simulink model "c960x4096_x14_7_r2013b_frb"  (R2013b)
settings: Solver=ode45  StartTime=0.0  StopTime=40960  RelTol=1e-3
undefined symbols (not defined in the file): sfp
libraries: xbsIndex_r4 x14620, casper_library_misc x61, dspsigops x32, casper_library_multipliers x24, simulink x18, xps_library x18
(part 36 of 79)

== system c960x4096_x14_7_r2013b_frb/ds_to_tgbe/mb_rd/XFER_5/GEN_R_ADDR_MUX_SEL ==
  MSYNC : Inport
  WE : Inport  Port=2
  NCHAN : Inport  Port=3
  9_bit_cntr : xbsIndex_r4/Counter  cnt_type=Free Running  cnt_to=Inf  operation=Up  start_count=0  cnt_by_val=1  arith_type=Unsigned  n_bits=9  bin_pt=0  load_pin=off  rst=on  en=on  explicit_period=on  period=1  dbl_ovrd=off  use_behavioral_HDL=off  implementation=Fabric  block_type=counter
  Concat : xbsIndex_r4/Concat  num_inputs=2  dbl_ovrd=off  block_type=concat
  DELAY_SEL : Subsystem
  Delay : xbsIndex_r4/Delay  rst=off  infoeditControl=Selection of Reset will increase slice count due to use of real FFs and instead of SRLs  en=off  latency=1  dbl_ovrd=off  reg_retiming=off  block_type=delay
  Logical : xbsIndex_r4/Logical  logical_function=OR  inputs=2  en=off  latency=0  precision=Full  arith_type=Unsigned  n_bits=16  bin_pt=0  align_bp=on  dbl_ovrd=off  block_type=logical
  Logical1 : xbsIndex_r4/Logical  logical_function=OR  inputs=2  en=off  latency=0  precision=Full  arith_type=Unsigned  n_bits=16  bin_pt=0  align_bp=on  dbl_ovrd=off  block_type=logical
  Logical2 : xbsIndex_r4/Logical  logical_function=OR  inputs=2  en=off  latency=0  precision=Full  arith_type=Unsigned  n_bits=16  bin_pt=0  align_bp=on  dbl_ovrd=off  block_type=logical
  Pad_3_MSBs : xbsIndex_r4/Constant  const=0  gui_display_data_type=Fixed-point  arith_type=Unsigned  n_bits=3  bin_pt=0  preci_type=Single  exp_width=8  frac_width=24  explicit_period=on  period=1  equ=P=C  opselect=C  inp2=PCIN>>17  opr=+  inp1=P  carry=CIN  dbl_ovrd=off  block_type=constant
  Register : xbsIndex_r4/Register  init=0  rst=on  en=off  dbl_ovrd=off  block_type=register
  Relational : xbsIndex_r4/Relational  mode=a=b  en=off  latency=0  dbl_ovrd=off  block_type=relational
  Slice_2_LSBs : xbsIndex_r4/Slice  nbits=2  boolean_output=off  mode=Lower Bit Location + Width  bit1=0  base1=MSB of Input  bit0=0  base0=LSB of Input  dbl_ovrd=off  block_type=slice
  Slice_7_MSBs : xbsIndex_r4/Slice  nbits=7  boolean_output=off  mode=Upper Bit Location + Width  bit1=0  base1=MSB of Input  bit0=0  base0=LSB of Input  dbl_ovrd=off  block_type=slice
  TERM_CNT : Subsystem
  edge_detect : Subsystem  AncestorBlock=casper_library_misc/edge_detect  mask(edge_detect){edge=Rising, polarity=Active High, x_in=[0 0.08 0.08 0.16 0.16 0.24 0.24 0.32 0.32 0.4], y_in=[-1 -1  1  1  1  1  1  1  1  1], x_out=[0.6 0.68 0.68 0.76 0.76 0.84 0.84 0.92 0.92 1], y_out=[-1 -1  1  1 -1 -1 -1 -1 -1 -1]}
      mask prompts: edge "Edge Type"; polarity "Output Polarity"; x_in "Input X Positions"; y_in "Input Y Positions"; x_out "Output X Positions"; y_out "Output Y Positions"
      mask help: Output is active for one-cycle after each edge of the specified type (i.e. rising, falling or both).
      mask init: same as c960x4096_x14_7_r2013b_frb/edge_detect2
      settings: AttributesFormatString=|
      | rising edges
      | active high
      mask Help: Output is active for one-cycle after each edge of the specified type (i.e. rising, falling, or both).  Latency is zero.
      mask TypeOptions edge: Rising | Falling | Both
      mask TypeOptions polarity: Active High | Active Low
      mask Display:
      | plot(x_in_num,0.5+y_in_num*0.2);
      | plot(x_out_num,0.5+y_out_num*0.2);
  R_ADDR : Outport
  MUX_SEL : Outport  Port=2
  wires:
  DELAY_SEL/1(TRIG) -> Logical/2
  edge_detect/1(out) -> DELAY_SEL/2(WE_PE)
  [NCHAN] -> DELAY_SEL/1(NCHAN)
  [WE] -> edge_detect/1(in)
  [MSYNC] -> Logical2/2
  Logical2/1 -> Register/2
  Register/1 -> 9_bit_cntr/2, Logical/1
  Logical/1 -> Register/1
  Delay/1 -> MUX_SEL/1
  NCHAN/1 -> [NCHAN]
  WE/1 -> [WE]
  MSYNC/1 -> [MSYNC]
  Slice_2_LSBs/1 -> Delay/1
  Concat/1 -> R_ADDR/1
  Relational/1 -> Logical1/1, Logical2/1
  Slice_7_MSBs/1 -> Concat/2
  Pad_3_MSBs/1 -> Concat/1
  [NCHAN] -> TERM_CNT/1(NCHAN)
  TERM_CNT/1(OUT) -> Relational/2
  [MSYNC] -> Logical1/2
  Logical1/1 -> 9_bit_cntr/1
  9_bit_cntr/1 -> Slice_7_MSBs/1, Slice_2_LSBs/1, Relational/1

== system c960x4096_x14_7_r2013b_frb/ds_to_tgbe/mb_rd/XFER_5/GEN_STB_EOF_W_COUNT ==
  MSYNC : Inport
  WE : Inport  Port=2
  NCHAN : Inport  Port=3
  2_RST : xbsIndex_r4/Constant  const=1027  gui_display_data_type=Fixed-point  arith_type=Unsigned  n_bits=11  bin_pt=0  preci_type=Single  exp_width=8  frac_width=24  explicit_period=on  period=1  equ=P=C  opselect=C  inp2=PCIN>>17  opr=+  inp1=P  carry=CIN  dbl_ovrd=off  block_type=constant
  A_LENGTH : Subsystem
  AddSub : xbsIndex_r4/AddSub  mode=Addition  use_carryin=off  use_carryout=off  en=off  latency=0  precision=Full  arith_type=Unsigned  n_bits=16  bin_pt=14  quantization=Truncate  overflow=Wrap  dbl_ovrd=off  use_behavioral_HDL=off  hw_selection=Fabric  pipelined=off  block_type=addsub
  B_LENGTH : Subsystem
  C_LENGTH : Subsystem
  Convert : xbsIndex_r4/Convert  gui_display_data_type=Fixed-point  arith_type=Unsigned  n_bits=1  bin_pt=0  float_type=Single  exp_bits=8  fraction_bits=24  quantization=Truncate  overflow=Wrap  en=off  latency=0  dbl_ovrd=off  pipeline=off  block_type=convert
  Convert1 : xbsIndex_r4/Convert  gui_display_data_type=Fixed-point  arith_type=Unsigned  n_bits=1  bin_pt=0  float_type=Single  exp_bits=8  fraction_bits=24  quantization=Truncate  overflow=Wrap  en=off  latency=0  dbl_ovrd=off  pipeline=off  block_type=convert
  Counter : xbsIndex_r4/Counter  cnt_type=Free Running  cnt_to=Inf  operation=Up  start_count=0  cnt_by_val=1  arith_type=Unsigned  n_bits=11  bin_pt=0  load_pin=off  rst=on  en=on  explicit_period=on  period=1  dbl_ovrd=off  use_behavioral_HDL=off  implementation=Fabric  block_type=counter
  Delay : xbsIndex_r4/Delay  rst=off  infoeditControl=Selection of Reset will increase slice count due to use of real FFs and instead of SRLs  en=off  latency=0  dbl_ovrd=off  reg_retiming=off  block_type=delay
  Delay1 : xbsIndex_r4/Delay  rst=off  infoeditControl=Selection of Reset will increase slice count due to use of real FFs and instead of SRLs  en=off  latency=1  dbl_ovrd=off  reg_retiming=off  block_type=delay
  Delay2 : xbsIndex_r4/Delay  rst=off  infoeditControl=Selection of Reset will increase slice count due to use of real FFs and instead of SRLs  en=off  latency=1  dbl_ovrd=off  reg_retiming=off  block_type=delay
  Delay3 : xbsIndex_r4/Delay  rst=off  infoeditControl=Selection of Reset will increase slice count due to use of real FFs and instead of SRLs  en=off  latency=2  dbl_ovrd=off  reg_retiming=off  block_type=delay
  Delay4 : xbsIndex_r4/Delay  rst=off  infoeditControl=Selection of Reset will increase slice count due to use of real FFs and instead of SRLs  en=off  latency=2  dbl_ovrd=off  reg_retiming=off  block_type=delay
  Delay5 : xbsIndex_r4/Delay  rst=off  infoeditControl=Selection of Reset will increase slice count due to use of real FFs and instead of SRLs  en=off  latency=1  dbl_ovrd=off  reg_retiming=off  block_type=delay
  Logical1 : xbsIndex_r4/Logical  logical_function=OR  inputs=2  en=off  latency=0  precision=Full  arith_type=Unsigned  n_bits=16  bin_pt=0  align_bp=on  dbl_ovrd=off  block_type=logical
  Mux : xbsIndex_r4/Mux  inputs=3  en=off  latency=0  precision=Full  arith_type=Unsigned  n_bits=16  bin_pt=14  quantization=Truncate  overflow=Wrap  dbl_ovrd=off  block_type=mux
  Pulse_Stretch : Subsystem
  Pulse_Stretch1 : Subsystem
  Pulse_Stretch2 : Subsystem
  Relational : xbsIndex_r4/Relational  mode=a>b  en=off  latency=0  dbl_ovrd=off  block_type=relational
  Relational1 : xbsIndex_r4/Relational  mode=a>b  en=off  latency=0  dbl_ovrd=off  block_type=relational
  Relational2 : xbsIndex_r4/Relational  mode=a=b  en=off  latency=0  dbl_ovrd=off  block_type=relational
  TO_DATA : Subsystem
  TO_FEC_ETC : Subsystem
  edge_detect : Subsystem  AncestorBlock=casper_library_misc/edge_detect  mask(edge_detect){edge=Falling, polarity=Active High, x_in=[0 0.08 0.08 0.16 0.16 0.24 0.24 0.32 0.32 0.4], y_in=[1  1 -1 -1 -1 -1 -1 -1 -1 -1], x_out=[0.6 0.68 0.68 0.76 0.76 0.84 0.84 0.92 0.92 1], y_out=[-1 -1  1  1 -1 -1 -1 -1 -1 -1]}
      mask prompts: edge "Edge Type"; polarity "Output Polarity"; x_in "Input X Positions"; y_in "Input Y Positions"; x_out "Output X Positions"; y_out "Output Y Positions"
      mask help: Output is active for one-cycle after each edge of the specified type (i.e. rising, falling or both).
      mask init: same as c960x4096_x14_7_r2013b_frb/edge_detect2
      settings: AttributesFormatString=|
      | falling edges
      | active high
      mask Help: Output is active for one-cycle after each edge of the specified type (i.e. rising, falling, or both).  Latency is zero.
      mask TypeOptions edge: Rising | Falling | Both
      mask TypeOptions polarity: Active High | Active Low
      mask Display:
      | plot(x_in_num,0.5+y_in_num*0.2);
      | plot(x_out_num,0.5+y_out_num*0.2);
  STB : Outport
  EOF : Outport  Port=2
  W_COUNT : Outport  Port=3
  wires:
  C_LENGTH/1(LEN) -> Pulse_Stretch2/3(LEN)
  B_LENGTH/1(LEN) -> Pulse_Stretch1/3(LEN)
  [MSYNC] -> Pulse_Stretch1/1(MSYNC), Pulse_Stretch2/1(MSYNC), Pulse_Stretch/1(MSYNC)
  [W_COUNT] -> Delay5/1
  [NCHAN] -> TO_FEC_ETC/1(NCHAN)
  TO_FEC_ETC/1(LEN) -> Relational1/2
  [NCHAN] -> TO_DATA/1(NCHAN)
  TO_DATA/1(LEN) -> Relational/2
  [NCHAN] -> C_LENGTH/1(NCHAN)
  [NCHAN] -> B_LENGTH/1(NCHAN)
  [NCHAN] -> A_LENGTH/1(NCHAN)
  A_LENGTH/1(LEN) -> Pulse_Stretch/3(LEN)
  NCHAN/1 -> [NCHAN]
  Delay2/1 -> [C]
  Delay1/1 -> [B]
  Delay/1 -> [A]
  [EOF] -> Delay4/1
  [STB] -> Delay3/1
  WE/1 -> edge_detect/1(in)
  MSYNC/1 -> [MSYNC], Logical1/1
  edge_detect/1(out) -> Pulse_Stretch2/2(IN), Pulse_Stretch1/2(IN), Pulse_Stretch/2(IN)
  Convert1/1 -> AddSub/2
  Convert/1 -> AddSub/1
  [STB] -> Counter/2
  [EOF] -> Logical1/2
  Relational2/1 -> [EOF]
  Mux/1 -> [STB]
  Logical1/1 -> Counter/1
  Relational1/1 -> Convert1/1
  Relational/1 -> Convert/1
  [W_COUNT] -> Relational2/1
  [W_COUNT] -> Relational1/1
  [W_COUNT] -> Relational/1
  2_RST/1 -> Relational2/2
  AddSub/1 -> [LEN_SEL], Mux/1
  [C] -> Mux/4
  [B] -> Mux/3
  [A] -> Mux/2
  Counter/1 -> [W_COUNT]
  Pulse_Stretch/1(OUT) -> Delay/1
  Pulse_Stretch2/1(OUT) -> Delay2/1
  Pulse_Stretch1/1(OUT) -> Delay1/1
  Delay3/1 -> STB/1
  Delay4/1 -> EOF/1
  Delay5/1 -> W_COUNT/1

== system c960x4096_x14_7_r2013b_frb/ds_to_tgbe/mb_rd/XFER_5/OUTPUT_MUX ==
  W_COUNT : Inport
  ENC_FC : Inport  Port=2
  DATA : Inport  Port=3
  FEC : Inport  Port=4
  IFG0 : Inport  Port=5
  IFG1 : Inport  Port=6
  ADV_2_STAATE_1 : xbsIndex_r4/Constant  const=0  gui_display_data_type=Fixed-point  arith_type=Unsigned  n_bits=11  bin_pt=0  preci_type=Single  exp_width=8  frac_width=24  explicit_period=on  period=1  equ=P=C  opselect=C  inp2=PCIN>>17  opr=+  inp1=P  carry=CIN  dbl_ovrd=off  block_type=constant
  ADV_2_STAATE_2 : xbsIndex_r4/Constant  const=1024  gui_display_data_type=Fixed-point  arith_type=Unsigned  n_bits=11  bin_pt=0  preci_type=Single  exp_width=8  frac_width=24  explicit_period=on  period=1  equ=P=C  opselect=C  inp2=PCIN>>17  opr=+  inp1=P  carry=CIN  dbl_ovrd=off  block_type=constant
  ADV_2_STAATE_3 : xbsIndex_r4/Constant  const=1025  gui_display_data_type=Fixed-point  arith_type=Unsigned  n_bits=11  bin_pt=0  preci_type=Single  exp_width=8  frac_width=24  explicit_period=on  period=1  equ=P=C  opselect=C  inp2=PCIN>>17  opr=+  inp1=P  carry=CIN  dbl_ovrd=off  block_type=constant
  ADV_2_STAATE_4 : xbsIndex_r4/Constant  const=1026  gui_display_data_type=Fixed-point  arith_type=Unsigned  n_bits=11  bin_pt=0  preci_type=Single  exp_width=8  frac_width=24  explicit_period=on  period=1  equ=P=C  opselect=C  inp2=PCIN>>17  opr=+  inp1=P  carry=CIN  dbl_ovrd=off  block_type=constant
  AddSub : xbsIndex_r4/AddSub  mode=Addition  use_carryin=off  use_carryout=off  en=off  latency=0  precision=Full  arith_type=Unsigned  n_bits=16  bin_pt=14  quantization=Truncate  overflow=Wrap  dbl_ovrd=off  use_behavioral_HDL=off  hw_selection=Fabric  pipelined=off  block_type=addsub
  AddSub1 : xbsIndex_r4/AddSub  mode=Addition  use_carryin=off  use_carryout=off  en=off  latency=0  precision=Full  arith_type=Unsigned  n_bits=16  bin_pt=14  quantization=Truncate  overflow=Wrap  dbl_ovrd=off  use_behavioral_HDL=off  hw_selection=Fabric  pipelined=off  block_type=addsub
  AddSub2 : xbsIndex_r4/AddSub  mode=Addition  use_carryin=off  use_carryout=off  en=off  latency=0  precision=Full  arith_type=Unsigned  n_bits=16  bin_pt=14  quantization=Truncate  overflow=Wrap  dbl_ovrd=off  use_behavioral_HDL=off  hw_selection=Fabric  pipelined=off  block_type=addsub
  Convert{,1..3} (4 alike) : xbsIndex_r4/Convert  gui_display_data_type=Fixed-point  arith_type=Unsigned  n_bits=1  bin_pt=0  float_type=Single  exp_bits=8  fraction_bits=24  quantization=Truncate  overflow=Wrap  en=off  latency=0  dbl_ovrd=off  pipeline=off  block_type=convert
  Delay2 : xbsIndex_r4/Delay  rst=off  infoeditControl=Selection of Reset will increase slice count due to use of real FFs and instead of SRLs  en=off  latency=1  dbl_ovrd=off  reg_retiming=off  block_type=delay
  Mux : xbsIndex_r4/Mux  inputs=5  en=off  latency=0  precision=Full  arith_type=Unsigned  n_bits=16  bin_pt=14  quantization=Truncate  overflow=Wrap  dbl_ovrd=off  block_type=mux
  Relational{1..4} (4 alike) : xbsIndex_r4/Relational  mode=a>b  en=off  latency=0  dbl_ovrd=off  block_type=relational
  DATA_OUT : Outport
  wires:
  Delay2/1 -> [DATA_OUT]
  AddSub2/1 -> Mux/1
  IFG1/1 -> [IFG1]
  IFG0/1 -> [IFG0]
  FEC/1 -> [FEC]
  [IFG1] -> Mux/6
  [IFG0] -> Mux/5
  [FEC] -> Mux/4
  [DATA] -> Mux/3
  DATA/1 -> [DATA]
  [ENC_FC] -> Mux/2
  ENC_FC/1 -> [ENC_FC]
  W_COUNT/1 -> [W_COUNT]
  AddSub1/1 -> AddSub2/2
  AddSub/1 -> AddSub2/1
  Convert3/1 -> AddSub1/2
  Convert2/1 -> AddSub1/1
  Convert1/1 -> AddSub/2
  Convert/1 -> AddSub/1
  Relational1/1 -> Convert/1
  Relational4/1 -> Convert3/1
  Relational3/1 -> Convert2/1
  Relational2/1 -> Convert1/1
  [W_COUNT] -> Relational4/1
  ADV_2_STAATE_4/1 -> Relational4/2
  [W_COUNT] -> Relational3/1
  ADV_2_STAATE_3/1 -> Relational3/2
  [W_COUNT] -> Relational2/1
  ADV_2_STAATE_2/1 -> Relational2/2
  [W_COUNT] -> Relational1/1
  ADV_2_STAATE_1/1 -> Relational1/2
  [DATA_OUT] -> DATA_OUT/1
  Mux/1 -> Delay2/1

== system c960x4096_x14_7_r2013b_frb/ds_to_tgbe/mb_rd/XFER_6/GEN_ENC_FC ==
  NODE_ID : Inport
  MSYNC : Inport  Port=2
  EOF : Inport  Port=3
  Concat : xbsIndex_r4/Concat  num_inputs=2  dbl_ovrd=off  block_type=concat
  Counter : xbsIndex_r4/Counter  cnt_type=Free Running  cnt_to=Inf  operation=Up  start_count=0  cnt_by_val=1  arith_type=Unsigned  n_bits=56  bin_pt=0  load_pin=off  rst=on  en=on  explicit_period=on  period=1  dbl_ovrd=off  use_behavioral_HDL=off  implementation=Fabric  block_type=counter
  ENC_FC : Outport
  wires:
  Concat/1 -> ENC_FC/1
  Counter/1 -> Concat/2
  NODE_ID/1 -> Concat/1
  EOF/1 -> Counter/2
  MSYNC/1 -> Counter/1

== system c960x4096_x14_7_r2013b_frb/ds_to_tgbe/mb_rd/XFER_6/GEN_R_ADDR_MUX_SEL ==
  MSYNC : Inport
  WE : Inport  Port=2
  NCHAN : Inport  Port=3
  9_bit_cntr : xbsIndex_r4/Counter  cnt_type=Free Running  cnt_to=Inf  operation=Up  start_count=0  cnt_by_val=1  arith_type=Unsigned  n_bits=9  bin_pt=0  load_pin=off  rst=on  en=on  explicit_period=on  period=1  dbl_ovrd=off  use_behavioral_HDL=off  implementation=Fabric  block_type=counter
  Concat : xbsIndex_r4/Concat  num_inputs=2  dbl_ovrd=off  block_type=concat
  DELAY_SEL : Subsystem
  Delay : xbsIndex_r4/Delay  rst=off  infoeditControl=Selection of Reset will increase slice count due to use of real FFs and instead of SRLs  en=off  latency=1  dbl_ovrd=off  reg_retiming=off  block_type=delay
  Logical : xbsIndex_r4/Logical  logical_function=OR  inputs=2  en=off  latency=0  precision=Full  arith_type=Unsigned  n_bits=16  bin_pt=0  align_bp=on  dbl_ovrd=off  block_type=logical
  Logical1 : xbsIndex_r4/Logical  logical_function=OR  inputs=2  en=off  latency=0  precision=Full  arith_type=Unsigned  n_bits=16  bin_pt=0  align_bp=on  dbl_ovrd=off  block_type=logical
  Logical2 : xbsIndex_r4/Logical  logical_function=OR  inputs=2  en=off  latency=0  precision=Full  arith_type=Unsigned  n_bits=16  bin_pt=0  align_bp=on  dbl_ovrd=off  block_type=logical
  Pad_3_MSBs : xbsIndex_r4/Constant  const=0  gui_display_data_type=Fixed-point  arith_type=Unsigned  n_bits=3  bin_pt=0  preci_type=Single  exp_width=8  frac_width=24  explicit_period=on  period=1  equ=P=C  opselect=C  inp2=PCIN>>17  opr=+  inp1=P  carry=CIN  dbl_ovrd=off  block_type=constant
  Register : xbsIndex_r4/Register  init=0  rst=on  en=off  dbl_ovrd=off  block_type=register
  Relational : xbsIndex_r4/Relational  mode=a=b  en=off  latency=0  dbl_ovrd=off  block_type=relational
  Slice_2_LSBs : xbsIndex_r4/Slice  nbits=2  boolean_output=off  mode=Lower Bit Location + Width  bit1=0  base1=MSB of Input  bit0=0  base0=LSB of Input  dbl_ovrd=off  block_type=slice
  Slice_7_MSBs : xbsIndex_r4/Slice  nbits=7  boolean_output=off  mode=Upper Bit Location + Width  bit1=0  base1=MSB of Input  bit0=0  base0=LSB of Input  dbl_ovrd=off  block_type=slice
  TERM_CNT : Subsystem
  edge_detect : Subsystem  AncestorBlock=casper_library_misc/edge_detect  mask(edge_detect){edge=Rising, polarity=Active High, x_in=[0 0.08 0.08 0.16 0.16 0.24 0.24 0.32 0.32 0.4], y_in=[-1 -1  1  1  1  1  1  1  1  1], x_out=[0.6 0.68 0.68 0.76 0.76 0.84 0.84 0.92 0.92 1], y_out=[-1 -1  1  1 -1 -1 -1 -1 -1 -1]}
      mask prompts: edge "Edge Type"; polarity "Output Polarity"; x_in "Input X Positions"; y_in "Input Y Positions"; x_out "Output X Positions"; y_out "Output Y Positions"
      mask help: Output is active for one-cycle after each edge of the specified type (i.e. rising, falling or both).
      mask init: same as c960x4096_x14_7_r2013b_frb/edge_detect2
      settings: AttributesFormatString=|
      | rising edges
      | active high
      mask Help: Output is active for one-cycle after each edge of the specified type (i.e. rising, falling, or both).  Latency is zero.
      mask TypeOptions edge: Rising | Falling | Both
      mask TypeOptions polarity: Active High | Active Low
      mask Display:
      | plot(x_in_num,0.5+y_in_num*0.2);
      | plot(x_out_num,0.5+y_out_num*0.2);
  R_ADDR : Outport
  MUX_SEL : Outport  Port=2
  wires:
  DELAY_SEL/1(TRIG) -> Logical/2
  edge_detect/1(out) -> DELAY_SEL/2(WE_PE)
  [NCHAN] -> DELAY_SEL/1(NCHAN)
  [WE] -> edge_detect/1(in)
  [MSYNC] -> Logical2/2
  Logical2/1 -> Register/2
  Register/1 -> 9_bit_cntr/2, Logical/1
  Logical/1 -> Register/1
  Delay/1 -> MUX_SEL/1
  NCHAN/1 -> [NCHAN]
  WE/1 -> [WE]
  MSYNC/1 -> [MSYNC]
  Slice_2_LSBs/1 -> Delay/1
  Concat/1 -> R_ADDR/1
  Relational/1 -> Logical1/1, Logical2/1
  Slice_7_MSBs/1 -> Concat/2
  Pad_3_MSBs/1 -> Concat/1
  [NCHAN] -> TERM_CNT/1(NCHAN)
  TERM_CNT/1(OUT) -> Relational/2
  [MSYNC] -> Logical1/2
  Logical1/1 -> 9_bit_cntr/1
  9_bit_cntr/1 -> Slice_7_MSBs/1, Slice_2_LSBs/1, Relational/1

== system c960x4096_x14_7_r2013b_frb/ds_to_tgbe/mb_rd/XFER_6/GEN_STB_EOF_W_COUNT ==
  MSYNC : Inport
  WE : Inport  Port=2
  NCHAN : Inport  Port=3
  2_RST : xbsIndex_r4/Constant  const=1027  gui_display_data_type=Fixed-point  arith_type=Unsigned  n_bits=11  bin_pt=0  preci_type=Single  exp_width=8  frac_width=24  explicit_period=on  period=1  equ=P=C  opselect=C  inp2=PCIN>>17  opr=+  inp1=P  carry=CIN  dbl_ovrd=off  block_type=constant
  A_LENGTH : Subsystem
  AddSub : xbsIndex_r4/AddSub  mode=Addition  use_carryin=off  use_carryout=off  en=off  latency=0  precision=Full  arith_type=Unsigned  n_bits=16  bin_pt=14  quantization=Truncate  overflow=Wrap  dbl_ovrd=off  use_behavioral_HDL=off  hw_selection=Fabric  pipelined=off  block_type=addsub
  B_LENGTH : Subsystem
  C_LENGTH : Subsystem
  Convert : xbsIndex_r4/Convert  gui_display_data_type=Fixed-point  arith_type=Unsigned  n_bits=1  bin_pt=0  float_type=Single  exp_bits=8  fraction_bits=24  quantization=Truncate  overflow=Wrap  en=off  latency=0  dbl_ovrd=off  pipeline=off  block_type=convert
  Convert1 : xbsIndex_r4/Convert  gui_display_data_type=Fixed-point  arith_type=Unsigned  n_bits=1  bin_pt=0  float_type=Single  exp_bits=8  fraction_bits=24  quantization=Truncate  overflow=Wrap  en=off  latency=0  dbl_ovrd=off  pipeline=off  block_type=convert
  Counter : xbsIndex_r4/Counter  cnt_type=Free Running  cnt_to=Inf  operation=Up  start_count=0  cnt_by_val=1  arith_type=Unsigned  n_bits=11  bin_pt=0  load_pin=off  rst=on  en=on  explicit_period=on  period=1  dbl_ovrd=off  use_behavioral_HDL=off  implementation=Fabric  block_type=counter
  Delay : xbsIndex_r4/Delay  rst=off  infoeditControl=Selection of Reset will increase slice count due to use of real FFs and instead of SRLs  en=off  latency=0  dbl_ovrd=off  reg_retiming=off  block_type=delay
  Delay1 : xbsIndex_r4/Delay  rst=off  infoeditControl=Selection of Reset will increase slice count due to use of real FFs and instead of SRLs  en=off  latency=1  dbl_ovrd=off  reg_retiming=off  block_type=delay
  Delay2 : xbsIndex_r4/Delay  rst=off  infoeditControl=Selection of Reset will increase slice count due to use of real FFs and instead of SRLs  en=off  latency=1  dbl_ovrd=off  reg_retiming=off  block_type=delay
  Delay3 : xbsIndex_r4/Delay  rst=off  infoeditControl=Selection of Reset will increase slice count due to use of real FFs and instead of SRLs  en=off  latency=2  dbl_ovrd=off  reg_retiming=off  block_type=delay
  Delay4 : xbsIndex_r4/Delay  rst=off  infoeditControl=Selection of Reset will increase slice count due to use of real FFs and instead of SRLs  en=off  latency=2  dbl_ovrd=off  reg_retiming=off  block_type=delay
  Delay5 : xbsIndex_r4/Delay  rst=off  infoeditControl=Selection of Reset will increase slice count due to use of real FFs and instead of SRLs  en=off  latency=1  dbl_ovrd=off  reg_retiming=off  block_type=delay
  Logical1 : xbsIndex_r4/Logical  logical_function=OR  inputs=2  en=off  latency=0  precision=Full  arith_type=Unsigned  n_bits=16  bin_pt=0  align_bp=on  dbl_ovrd=off  block_type=logical
  Mux : xbsIndex_r4/Mux  inputs=3  en=off  latency=0  precision=Full  arith_type=Unsigned  n_bits=16  bin_pt=14  quantization=Truncate  overflow=Wrap  dbl_ovrd=off  block_type=mux
  Pulse_Stretch : Subsystem
  Pulse_Stretch1 : Subsystem
  Pulse_Stretch2 : Subsystem
  Relational : xbsIndex_r4/Relational  mode=a>b  en=off  latency=0  dbl_ovrd=off  block_type=relational
  Relational1 : xbsIndex_r4/Relational  mode=a>b  en=off  latency=0  dbl_ovrd=off  block_type=relational
  Relational2 : xbsIndex_r4/Relational  mode=a=b  en=off  latency=0  dbl_ovrd=off  block_type=relational
  TO_DATA : Subsystem
  TO_FEC_ETC : Subsystem
  edge_detect : Subsystem  AncestorBlock=casper_library_misc/edge_detect  mask(edge_detect){edge=Falling, polarity=Active High, x_in=[0 0.08 0.08 0.16 0.16 0.24 0.24 0.32 0.32 0.4], y_in=[1  1 -1 -1 -1 -1 -1 -1 -1 -1], x_out=[0.6 0.68 0.68 0.76 0.76 0.84 0.84 0.92 0.92 1], y_out=[-1 -1  1  1 -1 -1 -1 -1 -1 -1]}
      mask prompts: edge "Edge Type"; polarity "Output Polarity"; x_in "Input X Positions"; y_in "Input Y Positions"; x_out "Output X Positions"; y_out "Output Y Positions"
      mask help: Output is active for one-cycle after each edge of the specified type (i.e. rising, falling or both).
      mask init: same as c960x4096_x14_7_r2013b_frb/edge_detect2
      settings: AttributesFormatString=|
      | falling edges
      | active high
      mask Help: Output is active for one-cycle after each edge of the specified type (i.e. rising, falling, or both).  Latency is zero.
      mask TypeOptions edge: Rising | Falling | Both
      mask TypeOptions polarity: Active High | Active Low
      mask Display:
      | plot(x_in_num,0.5+y_in_num*0.2);
      | plot(x_out_num,0.5+y_out_num*0.2);
  STB : Outport
  EOF : Outport  Port=2
  W_COUNT : Outport  Port=3
  wires:
  C_LENGTH/1(LEN) -> Pulse_Stretch2/3(LEN)
  B_LENGTH/1(LEN) -> Pulse_Stretch1/3(LEN)
  [MSYNC] -> Pulse_Stretch1/1(MSYNC), Pulse_Stretch2/1(MSYNC), Pulse_Stretch/1(MSYNC)
  [W_COUNT] -> Delay5/1
  [NCHAN] -> TO_FEC_ETC/1(NCHAN)
  TO_FEC_ETC/1(LEN) -> Relational1/2
  [NCHAN] -> TO_DATA/1(NCHAN)
  TO_DATA/1(LEN) -> Relational/2
  [NCHAN] -> C_LENGTH/1(NCHAN)
  [NCHAN] -> B_LENGTH/1(NCHAN)
  [NCHAN] -> A_LENGTH/1(NCHAN)
  A_LENGTH/1(LEN) -> Pulse_Stretch/3(LEN)
  NCHAN/1 -> [NCHAN]
  Delay2/1 -> [C]
  Delay1/1 -> [B]
  Delay/1 -> [A]
  [EOF] -> Delay4/1
  [STB] -> Delay3/1
  WE/1 -> edge_detect/1(in)
  MSYNC/1 -> [MSYNC], Logical1/1
  edge_detect/1(out) -> Pulse_Stretch2/2(IN), Pulse_Stretch1/2(IN), Pulse_Stretch/2(IN)
  Convert1/1 -> AddSub/2
  Convert/1 -> AddSub/1
  [STB] -> Counter/2
  [EOF] -> Logical1/2
  Relational2/1 -> [EOF]
  Mux/1 -> [STB]
  Logical1/1 -> Counter/1
  Relational1/1 -> Convert1/1
  Relational/1 -> Convert/1
  [W_COUNT] -> Relational2/1
  [W_COUNT] -> Relational1/1
  [W_COUNT] -> Relational/1
  2_RST/1 -> Relational2/2
  AddSub/1 -> [LEN_SEL], Mux/1
  [C] -> Mux/4
  [B] -> Mux/3
  [A] -> Mux/2
  Counter/1 -> [W_COUNT]
  Pulse_Stretch/1(OUT) -> Delay/1
  Pulse_Stretch2/1(OUT) -> Delay2/1
  Pulse_Stretch1/1(OUT) -> Delay1/1
  Delay3/1 -> STB/1
  Delay4/1 -> EOF/1
  Delay5/1 -> W_COUNT/1

== system c960x4096_x14_7_r2013b_frb/ds_to_tgbe/mb_rd/XFER_6/OUTPUT_MUX ==
  W_COUNT : Inport
  ENC_FC : Inport  Port=2
  DATA : Inport  Port=3
  FEC : Inport  Port=4
  IFG0 : Inport  Port=5
  IFG1 : Inport  Port=6
  ADV_2_STAATE_1 : xbsIndex_r4/Constant  const=0  gui_display_data_type=Fixed-point  arith_type=Unsigned  n_bits=11  bin_pt=0  preci_type=Single  exp_width=8  frac_width=24  explicit_period=on  period=1  equ=P=C  opselect=C  inp2=PCIN>>17  opr=+  inp1=P  carry=CIN  dbl_ovrd=off  block_type=constant
  ADV_2_STAATE_2 : xbsIndex_r4/Constant  const=1024  gui_display_data_type=Fixed-point  arith_type=Unsigned  n_bits=11  bin_pt=0  preci_type=Single  exp_width=8  frac_width=24  explicit_period=on  period=1  equ=P=C  opselect=C  inp2=PCIN>>17  opr=+  inp1=P  carry=CIN  dbl_ovrd=off  block_type=constant
  ADV_2_STAATE_3 : xbsIndex_r4/Constant  const=1025  gui_display_data_type=Fixed-point  arith_type=Unsigned  n_bits=11  bin_pt=0  preci_type=Single  exp_width=8  frac_width=24  explicit_period=on  period=1  equ=P=C  opselect=C  inp2=PCIN>>17  opr=+  inp1=P  carry=CIN  dbl_ovrd=off  block_type=constant
  ADV_2_STAATE_4 : xbsIndex_r4/Constant  const=1026  gui_display_data_type=Fixed-point  arith_type=Unsigned  n_bits=11  bin_pt=0  preci_type=Single  exp_width=8  frac_width=24  explicit_period=on  period=1  equ=P=C  opselect=C  inp2=PCIN>>17  opr=+  inp1=P  carry=CIN  dbl_ovrd=off  block_type=constant
  AddSub : xbsIndex_r4/AddSub  mode=Addition  use_carryin=off  use_carryout=off  en=off  latency=0  precision=Full  arith_type=Unsigned  n_bits=16  bin_pt=14  quantization=Truncate  overflow=Wrap  dbl_ovrd=off  use_behavioral_HDL=off  hw_selection=Fabric  pipelined=off  block_type=addsub
  AddSub1 : xbsIndex_r4/AddSub  mode=Addition  use_carryin=off  use_carryout=off  en=off  latency=0  precision=Full  arith_type=Unsigned  n_bits=16  bin_pt=14  quantization=Truncate  overflow=Wrap  dbl_ovrd=off  use_behavioral_HDL=off  hw_selection=Fabric  pipelined=off  block_type=addsub
  AddSub2 : xbsIndex_r4/AddSub  mode=Addition  use_carryin=off  use_carryout=off  en=off  latency=0  precision=Full  arith_type=Unsigned  n_bits=16  bin_pt=14  quantization=Truncate  overflow=Wrap  dbl_ovrd=off  use_behavioral_HDL=off  hw_selection=Fabric  pipelined=off  block_type=addsub
  Convert{,1..3} (4 alike) : xbsIndex_r4/Convert  gui_display_data_type=Fixed-point  arith_type=Unsigned  n_bits=1  bin_pt=0  float_type=Single  exp_bits=8  fraction_bits=24  quantization=Truncate  overflow=Wrap  en=off  latency=0  dbl_ovrd=off  pipeline=off  block_type=convert
  Delay2 : xbsIndex_r4/Delay  rst=off  infoeditControl=Selection of Reset will increase slice count due to use of real FFs and instead of SRLs  en=off  latency=1  dbl_ovrd=off  reg_retiming=off  block_type=delay
  Mux : xbsIndex_r4/Mux  inputs=5  en=off  latency=0  precision=Full  arith_type=Unsigned  n_bits=16  bin_pt=14  quantization=Truncate  overflow=Wrap  dbl_ovrd=off  block_type=mux
  Relational{1..4} (4 alike) : xbsIndex_r4/Relational  mode=a>b  en=off  latency=0  dbl_ovrd=off  block_type=relational
  DATA_OUT : Outport
  wires:
  Delay2/1 -> [DATA_OUT]
  AddSub2/1 -> Mux/1
  IFG1/1 -> [IFG1]
  IFG0/1 -> [IFG0]
  FEC/1 -> [FEC]
  [IFG1] -> Mux/6
  [IFG0] -> Mux/5
  [FEC] -> Mux/4
  [DATA] -> Mux/3
  DATA/1 -> [DATA]
  [ENC_FC] -> Mux/2
  ENC_FC/1 -> [ENC_FC]
  W_COUNT/1 -> [W_COUNT]
  AddSub1/1 -> AddSub2/2
  AddSub/1 -> AddSub2/1
  Convert3/1 -> AddSub1/2
  Convert2/1 -> AddSub1/1
  Convert1/1 -> AddSub/2
  Convert/1 -> AddSub/1
  Relational1/1 -> Convert/1
  Relational4/1 -> Convert3/1
  Relational3/1 -> Convert2/1
  Relational2/1 -> Convert1/1
  [W_COUNT] -> Relational4/1
  ADV_2_STAATE_4/1 -> Relational4/2
  [W_COUNT] -> Relational3/1
  ADV_2_STAATE_3/1 -> Relational3/2
  [W_COUNT] -> Relational2/1
  ADV_2_STAATE_2/1 -> Relational2/2
  [W_COUNT] -> Relational1/1
  ADV_2_STAATE_1/1 -> Relational1/2
  [DATA_OUT] -> DATA_OUT/1
  Mux/1 -> Delay2/1

== system c960x4096_x14_7_r2013b_frb/ds_to_tgbe/mb_rd/XFER_7/GEN_ENC_FC ==
  NODE_ID : Inport
  MSYNC : Inport  Port=2
  EOF : Inport  Port=3
  Concat : xbsIndex_r4/Concat  num_inputs=2  dbl_ovrd=off  block_type=concat
  Counter : xbsIndex_r4/Counter  cnt_type=Free Running  cnt_to=Inf  operation=Up  start_count=0  cnt_by_val=1  arith_type=Unsigned  n_bits=56  bin_pt=0  load_pin=off  rst=on  en=on  explicit_period=on  period=1  dbl_ovrd=off  use_behavioral_HDL=off  implementation=Fabric  block_type=counter
  ENC_FC : Outport
  wires:
  Concat/1 -> ENC_FC/1
  Counter/1 -> Concat/2
  NODE_ID/1 -> Concat/1
  EOF/1 -> Counter/2
  MSYNC/1 -> Counter/1

== system c960x4096_x14_7_r2013b_frb/ds_to_tgbe/mb_rd/XFER_7/GEN_R_ADDR_MUX_SEL ==
  MSYNC : Inport
  WE : Inport  Port=2
  NCHAN : Inport  Port=3
  9_bit_cntr : xbsIndex_r4/Counter  cnt_type=Free Running  cnt_to=Inf  operation=Up  start_count=0  cnt_by_val=1  arith_type=Unsigned  n_bits=9  bin_pt=0  load_pin=off  rst=on  en=on  explicit_period=on  period=1  dbl_ovrd=off  use_behavioral_HDL=off  implementation=Fabric  block_type=counter
  Concat : xbsIndex_r4/Concat  num_inputs=2  dbl_ovrd=off  block_type=concat
  DELAY_SEL : Subsystem
  Delay : xbsIndex_r4/Delay  rst=off  infoeditControl=Selection of Reset will increase slice count due to use of real FFs and instead of SRLs  en=off  latency=1  dbl_ovrd=off  reg_retiming=off  block_type=delay
  Logical : xbsIndex_r4/Logical  logical_function=OR  inputs=2  en=off  latency=0  precision=Full  arith_type=Unsigned  n_bits=16  bin_pt=0  align_bp=on  dbl_ovrd=off  block_type=logical
  Logical1 : xbsIndex_r4/Logical  logical_function=OR  inputs=2  en=off  latency=0  precision=Full  arith_type=Unsigned  n_bits=16  bin_pt=0  align_bp=on  dbl_ovrd=off  block_type=logical
  Logical2 : xbsIndex_r4/Logical  logical_function=OR  inputs=2  en=off  latency=0  precision=Full  arith_type=Unsigned  n_bits=16  bin_pt=0  align_bp=on  dbl_ovrd=off  block_type=logical
  Pad_3_MSBs : xbsIndex_r4/Constant  const=0  gui_display_data_type=Fixed-point  arith_type=Unsigned  n_bits=3  bin_pt=0  preci_type=Single  exp_width=8  frac_width=24  explicit_period=on  period=1  equ=P=C  opselect=C  inp2=PCIN>>17  opr=+  inp1=P  carry=CIN  dbl_ovrd=off  block_type=constant
  Register : xbsIndex_r4/Register  init=0  rst=on  en=off  dbl_ovrd=off  block_type=register
  Relational : xbsIndex_r4/Relational  mode=a=b  en=off  latency=0  dbl_ovrd=off  block_type=relational
  Slice_2_LSBs : xbsIndex_r4/Slice  nbits=2  boolean_output=off  mode=Lower Bit Location + Width  bit1=0  base1=MSB of Input  bit0=0  base0=LSB of Input  dbl_ovrd=off  block_type=slice
  Slice_7_MSBs : xbsIndex_r4/Slice  nbits=7  boolean_output=off  mode=Upper Bit Location + Width  bit1=0  base1=MSB of Input  bit0=0  base0=LSB of Input  dbl_ovrd=off  block_type=slice
  TERM_CNT : Subsystem
  edge_detect : Subsystem  AncestorBlock=casper_library_misc/edge_detect  mask(edge_detect){edge=Rising, polarity=Active High, x_in=[0 0.08 0.08 0.16 0.16 0.24 0.24 0.32 0.32 0.4], y_in=[-1 -1  1  1  1  1  1  1  1  1], x_out=[0.6 0.68 0.68 0.76 0.76 0.84 0.84 0.92 0.92 1], y_out=[-1 -1  1  1 -1 -1 -1 -1 -1 -1]}
      mask prompts: edge "Edge Type"; polarity "Output Polarity"; x_in "Input X Positions"; y_in "Input Y Positions"; x_out "Output X Positions"; y_out "Output Y Positions"
      mask help: Output is active for one-cycle after each edge of the specified type (i.e. rising, falling or both).
      mask init: same as c960x4096_x14_7_r2013b_frb/edge_detect2
      settings: AttributesFormatString=|
      | rising edges
      | active high
      mask Help: Output is active for one-cycle after each edge of the specified type (i.e. rising, falling, or both).  Latency is zero.
      mask TypeOptions edge: Rising | Falling | Both
      mask TypeOptions polarity: Active High | Active Low
      mask Display:
      | plot(x_in_num,0.5+y_in_num*0.2);
      | plot(x_out_num,0.5+y_out_num*0.2);
  R_ADDR : Outport
  MUX_SEL : Outport  Port=2
  wires:
  DELAY_SEL/1(TRIG) -> Logical/2
  edge_detect/1(out) -> DELAY_SEL/2(WE_PE)
  [NCHAN] -> DELAY_SEL/1(NCHAN)
  [WE] -> edge_detect/1(in)
  [MSYNC] -> Logical2/2
  Logical2/1 -> Register/2
  Register/1 -> 9_bit_cntr/2, Logical/1
  Logical/1 -> Register/1
  Delay/1 -> MUX_SEL/1
  NCHAN/1 -> [NCHAN]
  WE/1 -> [WE]
  MSYNC/1 -> [MSYNC]
  Slice_2_LSBs/1 -> Delay/1
  Concat/1 -> R_ADDR/1
  Relational/1 -> Logical1/1, Logical2/1
  Slice_7_MSBs/1 -> Concat/2
  Pad_3_MSBs/1 -> Concat/1
  [NCHAN] -> TERM_CNT/1(NCHAN)
  TERM_CNT/1(OUT) -> Relational/2
  [MSYNC] -> Logical1/2
  Logical1/1 -> 9_bit_cntr/1
  9_bit_cntr/1 -> Slice_7_MSBs/1, Slice_2_LSBs/1, Relational/1

== system c960x4096_x14_7_r2013b_frb/ds_to_tgbe/mb_rd/XFER_7/GEN_STB_EOF_W_COUNT ==
  MSYNC : Inport
  WE : Inport  Port=2
  NCHAN : Inport  Port=3
  2_RST : xbsIndex_r4/Constant  const=1027  gui_display_data_type=Fixed-point  arith_type=Unsigned  n_bits=11  bin_pt=0  preci_type=Single  exp_width=8  frac_width=24  explicit_period=on  period=1  equ=P=C  opselect=C  inp2=PCIN>>17  opr=+  inp1=P  carry=CIN  dbl_ovrd=off  block_type=constant
  A_LENGTH : Subsystem
  AddSub : xbsIndex_r4/AddSub  mode=Addition  use_carryin=off  use_carryout=off  en=off  latency=0  precision=Full  arith_type=Unsigned  n_bits=16  bin_pt=14  quantization=Truncate  overflow=Wrap  dbl_ovrd=off  use_behavioral_HDL=off  hw_selection=Fabric  pipelined=off  block_type=addsub
  B_LENGTH : Subsystem
  C_LENGTH : Subsystem
  Convert : xbsIndex_r4/Convert  gui_display_data_type=Fixed-point  arith_type=Unsigned  n_bits=1  bin_pt=0  float_type=Single  exp_bits=8  fraction_bits=24  quantization=Truncate  overflow=Wrap  en=off  latency=0  dbl_ovrd=off  pipeline=off  block_type=convert
  Convert1 : xbsIndex_r4/Convert  gui_display_data_type=Fixed-point  arith_type=Unsigned  n_bits=1  bin_pt=0  float_type=Single  exp_bits=8  fraction_bits=24  quantization=Truncate  overflow=Wrap  en=off  latency=0  dbl_ovrd=off  pipeline=off  block_type=convert
  Counter : xbsIndex_r4/Counter  cnt_type=Free Running  cnt_to=Inf  operation=Up  start_count=0  cnt_by_val=1  arith_type=Unsigned  n_bits=11  bin_pt=0  load_pin=off  rst=on  en=on  explicit_period=on  period=1  dbl_ovrd=off  use_behavioral_HDL=off  implementation=Fabric  block_type=counter
  Delay : xbsIndex_r4/Delay  rst=off  infoeditControl=Selection of Reset will increase slice count due to use of real FFs and instead of SRLs  en=off  latency=0  dbl_ovrd=off  reg_retiming=off  block_type=delay
  Delay1 : xbsIndex_r4/Delay  rst=off  infoeditControl=Selection of Reset will increase slice count due to use of real FFs and instead of SRLs  en=off  latency=1  dbl_ovrd=off  reg_retiming=off  block_type=delay
  Delay2 : xbsIndex_r4/Delay  rst=off  infoeditControl=Selection of Reset will increase slice count due to use of real FFs and instead of SRLs  en=off  latency=1  dbl_ovrd=off  reg_retiming=off  block_type=delay
  Delay3 : xbsIndex_r4/Delay  rst=off  infoeditControl=Selection of Reset will increase slice count due to use of real FFs and instead of SRLs  en=off  latency=2  dbl_ovrd=off  reg_retiming=off  block_type=delay
  Delay4 : xbsIndex_r4/Delay  rst=off  infoeditControl=Selection of Reset will increase slice count due to use of real FFs and instead of SRLs  en=off  latency=2  dbl_ovrd=off  reg_retiming=off  block_type=delay
  Delay5 : xbsIndex_r4/Delay  rst=off  infoeditControl=Selection of Reset will increase slice count due to use of real FFs and instead of SRLs  en=off  latency=1  dbl_ovrd=off  reg_retiming=off  block_type=delay
  Logical1 : xbsIndex_r4/Logical  logical_function=OR  inputs=2  en=off  latency=0  precision=Full  arith_type=Unsigned  n_bits=16  bin_pt=0  align_bp=on  dbl_ovrd=off  block_type=logical
  Mux : xbsIndex_r4/Mux  inputs=3  en=off  latency=0  precision=Full  arith_type=Unsigned  n_bits=16  bin_pt=14  quantization=Truncate  overflow=Wrap  dbl_ovrd=off  block_type=mux
  Pulse_Stretch : Subsystem
  Pulse_Stretch1 : Subsystem
  Pulse_Stretch2 : Subsystem
  Relational : xbsIndex_r4/Relational  mode=a>b  en=off  latency=0  dbl_ovrd=off  block_type=relational
  Relational1 : xbsIndex_r4/Relational  mode=a>b  en=off  latency=0  dbl_ovrd=off  block_type=relational
  Relational2 : xbsIndex_r4/Relational  mode=a=b  en=off  latency=0  dbl_ovrd=off  block_type=relational
  TO_DATA : Subsystem
  TO_FEC_ETC : Subsystem
  edge_detect : Subsystem  AncestorBlock=casper_library_misc/edge_detect  mask(edge_detect){edge=Falling, polarity=Active High, x_in=[0 0.08 0.08 0.16 0.16 0.24 0.24 0.32 0.32 0.4], y_in=[1  1 -1 -1 -1 -1 -1 -1 -1 -1], x_out=[0.6 0.68 0.68 0.76 0.76 0.84 0.84 0.92 0.92 1], y_out=[-1 -1  1  1 -1 -1 -1 -1 -1 -1]}
      mask prompts: edge "Edge Type"; polarity "Output Polarity"; x_in "Input X Positions"; y_in "Input Y Positions"; x_out "Output X Positions"; y_out "Output Y Positions"
      mask help: Output is active for one-cycle after each edge of the specified type (i.e. rising, falling or both).
      mask init: same as c960x4096_x14_7_r2013b_frb/edge_detect2
      settings: AttributesFormatString=|
      | falling edges
      | active high
      mask Help: Output is active for one-cycle after each edge of the specified type (i.e. rising, falling, or both).  Latency is zero.
      mask TypeOptions edge: Rising | Falling | Both
      mask TypeOptions polarity: Active High | Active Low
      mask Display:
      | plot(x_in_num,0.5+y_in_num*0.2);
      | plot(x_out_num,0.5+y_out_num*0.2);
  STB : Outport
  EOF : Outport  Port=2
  W_COUNT : Outport  Port=3
  wires:
  C_LENGTH/1(LEN) -> Pulse_Stretch2/3(LEN)
  B_LENGTH/1(LEN) -> Pulse_Stretch1/3(LEN)
  [MSYNC] -> Pulse_Stretch1/1(MSYNC), Pulse_Stretch2/1(MSYNC), Pulse_Stretch/1(MSYNC)
  [W_COUNT] -> Delay5/1
  [NCHAN] -> TO_FEC_ETC/1(NCHAN)
  TO_FEC_ETC/1(LEN) -> Relational1/2
  [NCHAN] -> TO_DATA/1(NCHAN)
  TO_DATA/1(LEN) -> Relational/2
  [NCHAN] -> C_LENGTH/1(NCHAN)
  [NCHAN] -> B_LENGTH/1(NCHAN)
  [NCHAN] -> A_LENGTH/1(NCHAN)
  A_LENGTH/1(LEN) -> Pulse_Stretch/3(LEN)
  NCHAN/1 -> [NCHAN]
  Delay2/1 -> [C]
  Delay1/1 -> [B]
  Delay/1 -> [A]
  [EOF] -> Delay4/1
  [STB] -> Delay3/1
  WE/1 -> edge_detect/1(in)
  MSYNC/1 -> [MSYNC], Logical1/1
  edge_detect/1(out) -> Pulse_Stretch2/2(IN), Pulse_Stretch1/2(IN), Pulse_Stretch/2(IN)
  Convert1/1 -> AddSub/2
  Convert/1 -> AddSub/1
  [STB] -> Counter/2
  [EOF] -> Logical1/2
  Relational2/1 -> [EOF]
  Mux/1 -> [STB]
  Logical1/1 -> Counter/1
  Relational1/1 -> Convert1/1
  Relational/1 -> Convert/1
  [W_COUNT] -> Relational2/1
  [W_COUNT] -> Relational1/1
  [W_COUNT] -> Relational/1
  2_RST/1 -> Relational2/2
  AddSub/1 -> [LEN_SEL], Mux/1
  [C] -> Mux/4
  [B] -> Mux/3
  [A] -> Mux/2
  Counter/1 -> [W_COUNT]
  Pulse_Stretch/1(OUT) -> Delay/1
  Pulse_Stretch2/1(OUT) -> Delay2/1
  Pulse_Stretch1/1(OUT) -> Delay1/1
  Delay3/1 -> STB/1
  Delay4/1 -> EOF/1
  Delay5/1 -> W_COUNT/1

== system c960x4096_x14_7_r2013b_frb/ds_to_tgbe/mb_rd/XFER_7/OUTPUT_MUX ==
  W_COUNT : Inport
  ENC_FC : Inport  Port=2
  DATA : Inport  Port=3
  FEC : Inport  Port=4
  IFG0 : Inport  Port=5
  IFG1 : Inport  Port=6
  ADV_2_STAATE_1 : xbsIndex_r4/Constant  const=0  gui_display_data_type=Fixed-point  arith_type=Unsigned  n_bits=11  bin_pt=0  preci_type=Single  exp_width=8  frac_width=24  explicit_period=on  period=1  equ=P=C  opselect=C  inp2=PCIN>>17  opr=+  inp1=P  carry=CIN  dbl_ovrd=off  block_type=constant
  ADV_2_STAATE_2 : xbsIndex_r4/Constant  const=1024  gui_display_data_type=Fixed-point  arith_type=Unsigned  n_bits=11  bin_pt=0  preci_type=Single  exp_width=8  frac_width=24  explicit_period=on  period=1  equ=P=C  opselect=C  inp2=PCIN>>17  opr=+  inp1=P  carry=CIN  dbl_ovrd=off  block_type=constant
  ADV_2_STAATE_3 : xbsIndex_r4/Constant  const=1025  gui_display_data_type=Fixed-point  arith_type=Unsigned  n_bits=11  bin_pt=0  preci_type=Single  exp_width=8  frac_width=24  explicit_period=on  period=1  equ=P=C  opselect=C  inp2=PCIN>>17  opr=+  inp1=P  carry=CIN  dbl_ovrd=off  block_type=constant
  ADV_2_STAATE_4 : xbsIndex_r4/Constant  const=1026  gui_display_data_type=Fixed-point  arith_type=Unsigned  n_bits=11  bin_pt=0  preci_type=Single  exp_width=8  frac_width=24  explicit_period=on  period=1  equ=P=C  opselect=C  inp2=PCIN>>17  opr=+  inp1=P  carry=CIN  dbl_ovrd=off  block_type=constant
  AddSub : xbsIndex_r4/AddSub  mode=Addition  use_carryin=off  use_carryout=off  en=off  latency=0  precision=Full  arith_type=Unsigned  n_bits=16  bin_pt=14  quantization=Truncate  overflow=Wrap  dbl_ovrd=off  use_behavioral_HDL=off  hw_selection=Fabric  pipelined=off  block_type=addsub
  AddSub1 : xbsIndex_r4/AddSub  mode=Addition  use_carryin=off  use_carryout=off  en=off  latency=0  precision=Full  arith_type=Unsigned  n_bits=16  bin_pt=14  quantization=Truncate  overflow=Wrap  dbl_ovrd=off  use_behavioral_HDL=off  hw_selection=Fabric  pipelined=off  block_type=addsub
  AddSub2 : xbsIndex_r4/AddSub  mode=Addition  use_carryin=off  use_carryout=off  en=off  latency=0  precision=Full  arith_type=Unsigned  n_bits=16  bin_pt=14  quantization=Truncate  overflow=Wrap  dbl_ovrd=off  use_behavioral_HDL=off  hw_selection=Fabric  pipelined=off  block_type=addsub
  Convert{,1..3} (4 alike) : xbsIndex_r4/Convert  gui_display_data_type=Fixed-point  arith_type=Unsigned  n_bits=1  bin_pt=0  float_type=Single  exp_bits=8  fraction_bits=24  quantization=Truncate  overflow=Wrap  en=off  latency=0  dbl_ovrd=off  pipeline=off  block_type=convert
  Delay2 : xbsIndex_r4/Delay  rst=off  infoeditControl=Selection of Reset will increase slice count due to use of real FFs and instead of SRLs  en=off  latency=1  dbl_ovrd=off  reg_retiming=off  block_type=delay
  Mux : xbsIndex_r4/Mux  inputs=5  en=off  latency=0  precision=Full  arith_type=Unsigned  n_bits=16  bin_pt=14  quantization=Truncate  overflow=Wrap  dbl_ovrd=off  block_type=mux
  Relational{1..4} (4 alike) : xbsIndex_r4/Relational  mode=a>b  en=off  latency=0  dbl_ovrd=off  block_type=relational
  DATA_OUT : Outport
  wires:
  Delay2/1 -> [DATA_OUT]
  AddSub2/1 -> Mux/1
  IFG1/1 -> [IFG1]
  IFG0/1 -> [IFG0]
  FEC/1 -> [FEC]
  [IFG1] -> Mux/6
  [IFG0] -> Mux/5
  [FEC] -> Mux/4
  [DATA] -> Mux/3
  DATA/1 -> [DATA]
  [ENC_FC] -> Mux/2
  ENC_FC/1 -> [ENC_FC]
  W_COUNT/1 -> [W_COUNT]
  AddSub1/1 -> AddSub2/2
  AddSub/1 -> AddSub2/1
  Convert3/1 -> AddSub1/2
  Convert2/1 -> AddSub1/1
  Convert1/1 -> AddSub/2
  Convert/1 -> AddSub/1
  Relational1/1 -> Convert/1
  Relational4/1 -> Convert3/1
  Relational3/1 -> Convert2/1
  Relational2/1 -> Convert1/1
  [W_COUNT] -> Relational4/1
  ADV_2_STAATE_4/1 -> Relational4/2
  [W_COUNT] -> Relational3/1
  ADV_2_STAATE_3/1 -> Relational3/2
  [W_COUNT] -> Relational2/1
  ADV_2_STAATE_2/1 -> Relational2/2
  [W_COUNT] -> Relational1/1
  ADV_2_STAATE_1/1 -> Relational1/2
  [DATA_OUT] -> DATA_OUT/1
  Mux/1 -> Delay2/1

== system c960x4096_x14_7_r2013b_frb/ds_to_tgbe/mb_wr/MB_WRITE_SLICES/ADDR_1 ==
  ADDR_CNT : Inport
  NO_LSB : xbsIndex_r4/Constant  const=0  gui_display_data_type=Fixed-point  arith_type=Unsigned  n_bits=10  bin_pt=0  preci_type=Single  exp_width=8  frac_width=24  explicit_period=on  period=1  equ=P=C  opselect=C  inp2=PCIN>>17  opr=+  inp1=P  carry=CIN  dbl_ovrd=off  block_type=constant
  Terminator : Terminator
  W_ADDR : Outport
  wires:
  NO_LSB/1 -> W_ADDR/1
  ADDR_CNT/1 -> Terminator/1

== system c960x4096_x14_7_r2013b_frb/ds_to_tgbe/mb_wr/MB_WRITE_SLICES/ADDR_128 ==
  ADDR_CNT : Inport
  Concat : xbsIndex_r4/Concat  num_inputs=2  dbl_ovrd=off  block_type=concat
  PAD_3_MSBs : xbsIndex_r4/Constant  const=0  gui_display_data_type=Fixed-point  arith_type=Unsigned  n_bits=3  bin_pt=0  preci_type=Single  exp_width=8  frac_width=24  explicit_period=off  period=1  equ=P=C  opselect=C  inp2=PCIN>>17  opr=+  inp1=P  carry=CIN  dbl_ovrd=off  block_type=constant
  Slice_7_LSBs : xbsIndex_r4/Slice  nbits=7  boolean_output=off  mode=Lower Bit Location + Width  bit1=0  base1=MSB of Input  bit0=0  base0=LSB of Input  dbl_ovrd=off  block_type=slice
  W_ADDR : Outport
  wires:
  Concat/1 -> W_ADDR/1
  Slice_7_LSBs/1 -> Concat/2
  PAD_3_MSBs/1 -> Concat/1
  ADDR_CNT/1 -> Slice_7_LSBs/1

== system c960x4096_x14_7_r2013b_frb/ds_to_tgbe/mb_wr/MB_WRITE_SLICES/ADDR_16 ==
  ADDR_CNT : Inport
  Concat : xbsIndex_r4/Concat  num_inputs=2  dbl_ovrd=off  block_type=concat
  PAD_6_MSBs : xbsIndex_r4/Constant  const=0  gui_display_data_type=Fixed-point  arith_type=Unsigned  n_bits=6  bin_pt=0  preci_type=Single  exp_width=8  frac_width=24  explicit_period=on  period=1  equ=P=C  opselect=C  inp2=PCIN>>17  opr=+  inp1=P  carry=CIN  dbl_ovrd=off  block_type=constant
  Slice_4_LSBs : xbsIndex_r4/Slice  nbits=4  boolean_output=off  mode=Lower Bit Location + Width  bit1=0  base1=MSB of Input  bit0=0  base0=LSB of Input  dbl_ovrd=off  block_type=slice
  W_ADDR : Outport
  wires:
  Concat/1 -> W_ADDR/1
  ADDR_CNT/1 -> Slice_4_LSBs/1
  Slice_4_LSBs/1 -> Concat/2
  PAD_6_MSBs/1 -> Concat/1

== system c960x4096_x14_7_r2013b_frb/ds_to_tgbe/mb_wr/MB_WRITE_SLICES/ADDR_2 ==
  ADDR_CNT : Inport
  Concat : xbsIndex_r4/Concat  num_inputs=2  dbl_ovrd=off  block_type=concat
  PAD_9_MSBs : xbsIndex_r4/Constant  const=0  gui_display_data_type=Fixed-point  arith_type=Unsigned  n_bits=9  bin_pt=0  preci_type=Single  exp_width=8  frac_width=24  explicit_period=on  period=1  equ=P=C  opselect=C  inp2=PCIN>>17  opr=+  inp1=P  carry=CIN  dbl_ovrd=off  block_type=constant
  Slice_LSB : xbsIndex_r4/Slice  nbits=1  boolean_output=off  mode=Lower Bit Location + Width  bit1=0  base1=MSB of Input  bit0=0  base0=LSB of Input  dbl_ovrd=off  block_type=slice
  W_ADDR : Outport
  wires:
  Concat/1 -> W_ADDR/1
  ADDR_CNT/1 -> Slice_LSB/1
  Slice_LSB/1 -> Concat/2
  PAD_9_MSBs/1 -> Concat/1

== system c960x4096_x14_7_r2013b_frb/ds_to_tgbe/mb_wr/MB_WRITE_SLICES/ADDR_32 ==
  ADDR_CNT : Inport
  Concat : xbsIndex_r4/Concat  num_inputs=2  dbl_ovrd=off  block_type=concat
  PAD_5_MSBs : xbsIndex_r4/Constant  const=0  gui_display_data_type=Fixed-point  arith_type=Unsigned  n_bits=5  bin_pt=0  preci_type=Single  exp_width=8  frac_width=24  explicit_period=on  period=1  equ=P=C  opselect=C  inp2=PCIN>>17  opr=+  inp1=P  carry=CIN  dbl_ovrd=off  block_type=constant
  Slice_5_LSBs : xbsIndex_r4/Slice  nbits=5  boolean_output=off  mode=Lower Bit Location + Width  bit1=0  base1=MSB of Input  bit0=0  base0=LSB of Input  dbl_ovrd=off  block_type=slice
  W_ADDR : Outport
  wires:
  Concat/1 -> W_ADDR/1
  ADDR_CNT/1 -> Slice_5_LSBs/1
  Slice_5_LSBs/1 -> Concat/2
  PAD_5_MSBs/1 -> Concat/1

== system c960x4096_x14_7_r2013b_frb/ds_to_tgbe/mb_wr/MB_WRITE_SLICES/ADDR_4 ==
  ADDR_CNT : Inport
  Concat : xbsIndex_r4/Concat  num_inputs=2  dbl_ovrd=off  block_type=concat
  PAD_8_MSBs : xbsIndex_r4/Constant  const=0  gui_display_data_type=Fixed-point  arith_type=Unsigned  n_bits=8  bin_pt=0  preci_type=Single  exp_width=8  frac_width=24  explicit_period=on  period=1  equ=P=C  opselect=C  inp2=PCIN>>17  opr=+  inp1=P  carry=CIN  dbl_ovrd=off  block_type=constant
  Slice_2_LSBs : xbsIndex_r4/Slice  nbits=2  boolean_output=off  mode=Lower Bit Location + Width  bit1=0  base1=MSB of Input  bit0=0  base0=LSB of Input  dbl_ovrd=off  block_type=slice
  W_ADDR : Outport
  wires:
  Concat/1 -> W_ADDR/1
  ADDR_CNT/1 -> Slice_2_LSBs/1
  Slice_2_LSBs/1 -> Concat/2
  PAD_8_MSBs/1 -> Concat/1

== system c960x4096_x14_7_r2013b_frb/ds_to_tgbe/mb_wr/MB_WRITE_SLICES/ADDR_64 ==
  ADDR_CNT : Inport
  Concat : xbsIndex_r4/Concat  num_inputs=2  dbl_ovrd=off  block_type=concat
  PAD_4_MSBs : xbsIndex_r4/Constant  const=0  gui_display_data_type=Fixed-point  arith_type=Unsigned  n_bits=4  bin_pt=0  preci_type=Single  exp_width=8  frac_width=24  explicit_period=on  period=1  equ=P=C  opselect=C  inp2=PCIN>>17  opr=+  inp1=P  carry=CIN  dbl_ovrd=off  block_type=constant
  Slice_6_LSBs : xbsIndex_r4/Slice  nbits=6  boolean_output=off  mode=Lower Bit Location + Width  bit1=0  base1=MSB of Input  bit0=0  base0=LSB of Input  dbl_ovrd=off  block_type=slice
  W_ADDR : Outport
  wires:
  Concat/1 -> W_ADDR/1
  ADDR_CNT/1 -> Slice_6_LSBs/1
  Slice_6_LSBs/1 -> Concat/2
  PAD_4_MSBs/1 -> Concat/1
